simulink model "model_2018b"  (R2018b)
settings: Solver=VariableStepAuto  StartTime=0.0  StopTime=1.0  RelTol=1e-3
values from neighbouring files (symbols this model uses):
  delta_t = 0.1    [Parallelized_Model_Call.m]    (also in constants_v1.mat)
  density_of_cf = 1550    [Model_Call.m]    (also in Parallelized_Model_Call.m = density_of_material; constants_v1.mat)
  density_of_foam = 64.07    [Model_Call.m]    (also in Parallelized_Model_Call.m; constants_v1.mat)
  f_t = 2.48    [Model_Call.m]    (also in Parallelized_Model_Call.m = thrust_12v(pwm == pwm_start); constants_v1.mat; solve_for_cruising_velocity.m = u(3))
  height = 0.45    [Model_Call.m]    (also in find_closest_height_for_given_area.m = u(3); find_wetted_surface_area.m = u(3))
  length_imp = 0.2    [Parallelized_Model_Call.m]    (also in constants_v1.mat)
  percent_of_hull_with_foam = 0.5    [Model_Call.m]    (also in Parallelized_Model_Call.m; constants_v1.mat)
  thickness_of_cf = 0.003    [Model_Call.m]    (also in Parallelized_Model_Call.m = thickness_of_material; constants_v1.mat)
  V_impact = sqrt(2*g*dropHeight)    [Parallelized_Model_Call.m]    (also in constants_v1.mat = 9.47114776571)
  water_density = 1000    [Model_Call.m]    (also in Parallelized_Model_Call.m; constants_v1.mat)
  water_viscosity = 0.001    [Model_Call.m]    (also in Parallelized_Model_Call.m; constants_v1.mat)
  weight_of_battery = 2    [Model_Call.m]    (also in Parallelized_Model_Call.m = battery_count * weight_of_battery_single)
  weight_of_frame = 3    [Model_Call.m]    (also in Parallelized_Model_Call.m; constants_v1.mat)
  weight_of_junction_box = 2    [Model_Call.m]    (also in Parallelized_Model_Call.m; constants_v1.mat)
  weight_of_motors = 0.344 * 4    (= 1.376)    [Model_Call.m]    (also in Parallelized_Model_Call.m; constants_v1.mat)
  weight_of_other_electronics = 2    [Model_Call.m]    (also in Parallelized_Model_Call.m; constants_v1.mat)
  weight_of_payload = 4.5    [Model_Call.m]    (also in Parallelized_Model_Call.m = 3; constants_v1.mat = 3)
  width = 0.15    [Model_Call.m]    (also in find_closest_height_for_given_area.m = u(2); find_wetted_surface_area.m = u(2))
  width_imp = 0.2    [Parallelized_Model_Call.m]    (also in constants_v1.mat)
settings Model: Creator=akulkarni  LastModifiedBy=Owner
settings DataIOCC: ReturnWorkspaceOutputs=on

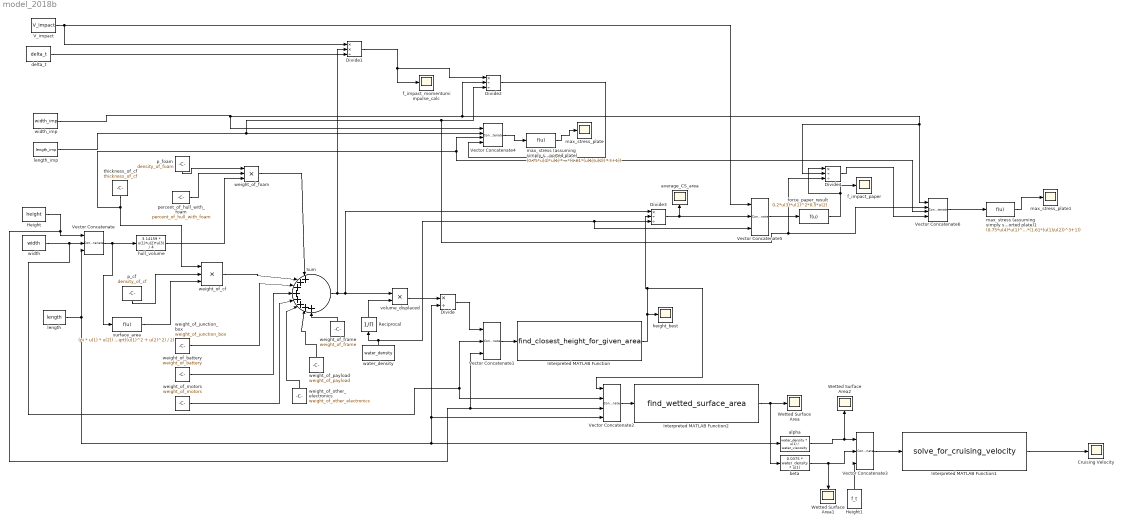
== system model_2018b ==
  Cruising Velocity : Scope
  Divide : Product  Inputs=*/
  Divide1 : Product  Inputs=**/
  Divide2 : Product  Inputs=*//
  Divide3 : Product  Inputs=*//
  Divide4 : Product  Inputs=*//
  Height : Constant  Value=height
  Height1 : Constant  Value=f_t
  Interpreted MATLAB Function : MATLABFcn  MATLABFcn=find_closest_height_for_given_area  OutputDimensions=1
  Interpreted MATLAB Function1 : MATLABFcn  MATLABFcn=solve_for_cruising_velocity  OutputDimensions=1
  Interpreted MATLAB Function2 : MATLABFcn  MATLABFcn=find_wetted_surface_area  OutputDimensions=1
  Reciprocal : Product  Inputs=/
  Sum : Sum  Inputs=|++++++++
  V_impact : Constant  Value=V_impact
  Vector Concatenate{,1,3,5} (4 alike) : Concatenate  NumInputs=3
  Vector Concatenate2 : Concatenate  NumInputs=4
  Vector Concatenate4 : Concatenate  NumInputs=4
  Vector Concatenate6 : Concatenate  NumInputs=4
  Wetted Surface Area : Scope
  Wetted Surface Area1 : Scope
  Wetted Surface Area2 : Scope
  alpha : Fcn  Expr=water_density * u(1) / water_viscosity
  average_CS_area : Scope
  beta : Fcn  Expr=0.0375 * water_density * u(1)
  delta_t : Constant  Value=delta_t
  f_impact_momentumimpulse_calc : Scope
  f_impact_paper : Scope
  force_paper_result : Fcn  Expr=0.2*u(3)*u(1)^2*0.5*u(2)
  height_best : Scope
  hull_volume : Fcn  Expr=3.14159 * u(1)*u(2)*u(3) / 4
  "length " : Constant  Value=length
  length_imp : Constant  Value=length_imp
  max_stress (assuming simply supported plate) : Fcn  Expr=(0.75*u(4)*u(1)^2)/(u(3)^2*(1.61*(u(1)/u(2))^3+1))
  max_stress (assuming simply supported plate)1 : Fcn  Expr=(0.75*u(4)*u(1)^2)/(u(3)^2*(1.61*(u(1)/u(2))^3+1))
  max_stress_plate : Scope
  max_stress_plate1 : Scope
  "p_cf " : Constant  Value=density_of_cf
  p_foam : Constant  Value=density_of_foam
  "percent_of_hull_with_foam " : Constant  Value=percent_of_hull_with_foam
  "surface_area " : Fcn  Expr=(pi * u(1) * u(2)) / 2 + pi * u(3) * sqrt((u(1)^2 + u(2)^2) / 2)
  thickness_of_cf : Constant  Value=thickness_of_cf
  volume_displaced : Product
  water_density : Constant  Value=water_density
  weight_of_battery : Constant  Value=weight_of_battery
  weight_of_cf : Product  Inputs=3
  weight_of_foam : Product  Inputs=3
  weight_of_frame : Constant  Value=weight_of_frame
  weight_of_junction_box : Constant  Value=weight_of_junction_box
  weight_of_motors : Constant  Value=weight_of_motors
  weight_of_other_electronics : Constant  Value=weight_of_other_electronics
  weight_of_payload : Constant  Value=weight_of_payload
  width : Constant  Value=width
  width_imp : Constant  Value=width_imp
  wires:
  p_foam/1 -> weight_of_foam/1
  "percent_of_hull_with_foam "/1 -> weight_of_foam/2
  Height/1 -> Vector Concatenate/1, Vector Concatenate1/3, Vector Concatenate2/3
  "length "/1 -> Vector Concatenate/3, alpha/1, Divide/2, Vector Concatenate2/4
  Vector Concatenate/1 -> "surface_area "/1, hull_volume/1
  hull_volume/1 -> weight_of_foam/3
  "surface_area "/1 -> weight_of_cf/3
  "p_cf "/1 -> weight_of_cf/2
  thickness_of_cf/1 -> weight_of_cf/1, Vector Concatenate4/3, Vector Concatenate6/3
  weight_of_foam/1 -> Sum/1
  weight_of_cf/1 -> Sum/2
  weight_of_junction_box/1 -> Sum/3
  weight_of_battery/1 -> Sum/4
  weight_of_motors/1 -> Sum/5
  weight_of_other_electronics/1 -> Sum/6
  Sum/1 -> Divide3/1, volume_displaced/1, Divide1/2
  water_density/1 -> Reciprocal/1, Vector Concatenate5/3, Divide3/3
  Reciprocal/1 -> volume_displaced/2
  volume_displaced/1 -> Divide/1
  Divide/1 -> Vector Concatenate1/1
  weight_of_frame/1 -> Sum/8
  weight_of_payload/1 -> Sum/7
  Vector Concatenate1/1 -> Interpreted MATLAB Function/1
  Interpreted MATLAB Function/1 -> Divide3/2, Vector Concatenate2/1, height_best/1
  width/1 -> Vector Concatenate2/2, Vector Concatenate1/2, Vector Concatenate/2
  Vector Concatenate2/1 -> Interpreted MATLAB Function2/1
  Interpreted MATLAB Function2/1 -> beta/1, Wetted Surface Area/1
  Vector Concatenate3/1 -> Interpreted MATLAB Function1/1
  alpha/1 -> Wetted Surface Area2/1, Vector Concatenate3/1
  beta/1 -> Vector Concatenate3/2, Wetted Surface Area1/1
  Height1/1 -> Vector Concatenate3/3
  Interpreted MATLAB Function1/1 -> Cruising Velocity/1
  V_impact/1 -> Divide1/1, Vector Concatenate5/1
  delta_t/1 -> Divide1/3
  Divide1/1 -> f_impact_momentumimpulse_calc/1, Divide2/1
  width_imp/1 -> Vector Concatenate4/1, Vector Concatenate6/1, Divide4/2, Divide2/2
  length_imp/1 -> Divide2/3, Vector Concatenate6/2, Divide4/3, Vector Concatenate4/2
  Vector Concatenate4/1 -> max_stress (assuming simply supported plate)/1
  Divide2/1 -> Vector Concatenate4/4
  max_stress (assuming simply supported plate)/1 -> max_stress_plate/1
  Divide3/1 -> Vector Concatenate5/2, average_CS_area/1
  Vector Concatenate5/1 -> force_paper_result/1
  Divide4/1 -> Vector Concatenate6/4
  Vector Concatenate6/1 -> max_stress (assuming simply supported plate)1/1
  max_stress (assuming simply supported plate)1/1 -> max_stress_plate1/1
  force_paper_result/1 -> f_impact_paper/1, Divide4/1
